simulink model "CranePID1"  (Simulink 5.0)
settings: Solver=ode5  SolverMode=SingleTasking  StartTime=0.0  StopTime=50.0  FixedStep=0.001  RelTol=1e-3
libraries: pci1711 x3
settings Model: LastModifiedBy=cedrics  ExtModeMexFile=rtwinext  ExtModeTrigMode=oneshot  ExtModeTrigDuration=100000  ExtModeLogAll=off  SimulationMode=external  LimitDataPoints=off  BlockReductionOpt=off  BooleanDataType=off  RTWSystemTargetFile=rtwinfbk.tlc  RTWTemplateMakefile=winfbktmf  RTWOptions="-aCCOptimize=1 -aEnforceIntegerDowncast=1 -aExtMode=1 -aFoldNonRolledExpr=1 -aForceParamTrailComments=0 -aGenerateComments=1 -aGenerateReport=0 -aIncDataTypeInIds=0 -aIncHierarchyInIds=0 -aInlineInvariantSignals=0 -aInlineParameters=0 -aInlinedPrmAccess=\"Literals\" -aLocalBlockOutputs=1 -aMaxRTWIdLen=31 -aPrefixModelToSubsysFcnNames=1 -aRTWVerbose=1 -aRebuildAll=0 -aRollThreshold=5 -aShowEliminatedStatements=1"

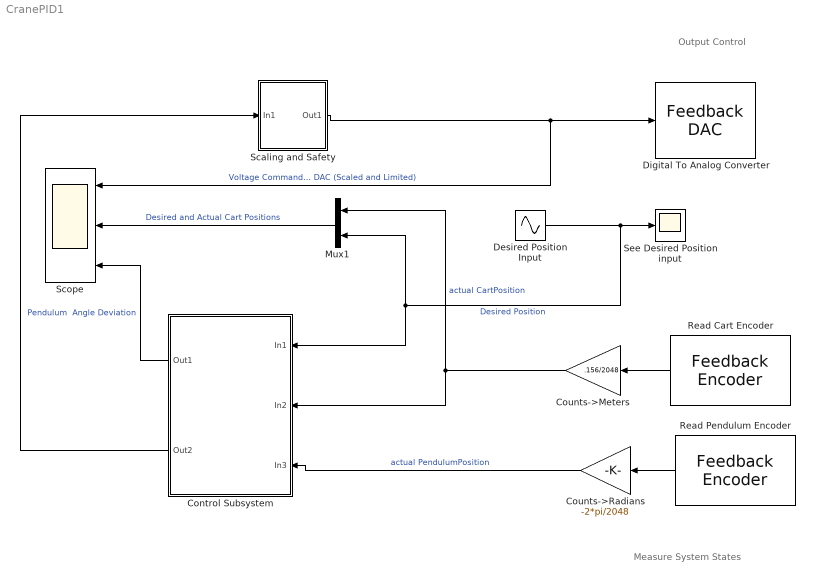
== system CranePID1 ==
  note: Measure System States
  note: Output Control
  Control Subsystem : Subsystem  Orientation=left
  Counts->Meters : Gain  Orientation=left  Gain=.156/2048  SaturateOnIntegerOverflow=on
  Counts->Radians : Gain  Orientation=left  Gain=-2*pi/2048  SaturateOnIntegerOverflow=on
  Desired Position Input : Sin  Amplitude=0.2  SampleTime=0
  "Digital To Analog Converter " : pci1711/Advantech  PCI1711 I//O Board Lib/Feedback DAC  channel=0  range=0  tsamp=0.001  hwAccess=on
  Mux1 : Mux  Orientation=left  Inputs=2
  Read Cart Encoder : pci1711/Advantech  PCI1711 I//O Board Lib/Feedback Encoder   Orientation=left  channel=0  offset=0  tsamp=0.001  hwAccess=on
  Read Pendulum Encoder : pci1711/Advantech  PCI1711 I//O Board Lib/Feedback Encoder   Orientation=left  channel=1  offset=-1024  tsamp=0.001  hwAccess=on
  Scaling and Safety : Subsystem
  Scope : Scope  NumInputPorts=3
      settings: TickLabels=on  TimeRange=50  YMin=-2.5~-0.3~-3.5  YMax=2.5~0.3~3.5  Decimation=10  SampleInput=on  SampleTime=0.01
  See Desired Position input : Scope
      settings: YMin=-0.75  YMax=1.5  SampleInput=on  SampleTime=0.1
  wires:
  Read Cart Encoder/1 -> Counts->Meters/1
  Counts->Meters/1 -> Mux1/1, Control Subsystem/2(In2)  "actual CartPosition"
  Counts->Radians/1 -> Control Subsystem/3(In3)  "actual PendulumPosition"
  Control Subsystem/2(Out2) -> Scaling and Safety/1(In1)
  Mux1/1 -> Scope/2  "Desired and Actual Cart Positions"
  Control Subsystem/1(Out1) -> Scope/3  "Pendulum  Angle Deviation"
  Read Pendulum Encoder/1 -> Counts->Radians/1
  Scaling and Safety/1(Out1) -> Scope/1, "Digital To Analog Converter "/1  "Voltage Command to DAC (Scaled and Limited)"
  Desired Position Input/1 -> Mux1/2, Control Subsystem/1(In1), See Desired Position input/1  "Desired Position"

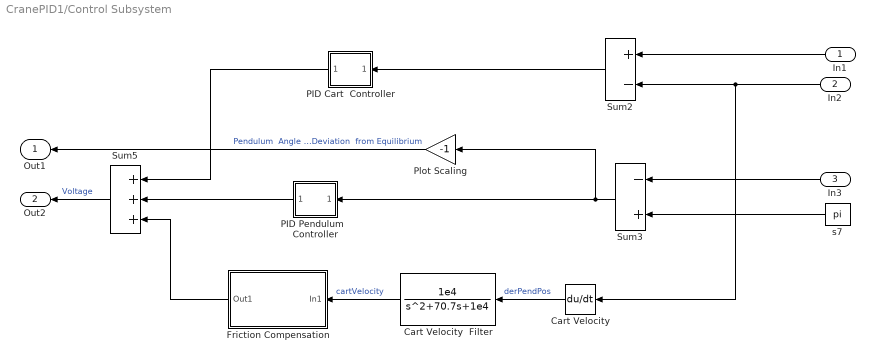
== system CranePID1/Control Subsystem ==
  In1 : Inport  Orientation=left
  In2 : Inport  Orientation=left  Port=2
  In3 : Inport  Orientation=left  Port=3
  Cart Velocity : Derivative  Orientation=left
  Cart Velocity  Filter : TransferFcn  Orientation=left  Numerator=[1e4]  Denominator=[1 70.7 1e4]
  Friction Compensation : Subsystem  Orientation=left  mask(linear){frictionCompNeg=.1, frictionCompPos=.1}
      mask prompts: frictionCompNeg "Friction Compensation Magnitude in Negative Direction"; frictionCompPos "Friction Compensation Magnitude in Positive Direction"
      mask Display: plot(0,0,100,100,[40,30,20],[87,85,80],[46,54,54,46,46],[90,90,80,80,90],[46,45,45,46,54,55,55,54,46],[78,80,90,91,91,90,80,78,78],[51,51,49,49],[78,10,10,78],[90,80,70,60],[70,80,85,88],[20,10],[80,70],[20,20,15],[73,80,80],[85,80,80],[80,80,74])
  PID Cart  Controller : Subsystem  Orientation=left  mask(PID Controller){@1=10, @2=1, @3=2}
      mask prompts: @1 "Proportional:"; @2 "Integral"; @3 "Derivative:"
      mask help:
      | Enter expressions for proportional, integral, and derivative terms.
      | P+I/s+Ds
      mask init:
      | P=@1; I=@2; D=@3;
      mask Help: This block implements a PID controller where parameters are entered for the Proportional, Integral and Derivative terms. Unmask this block to see how it works. The derivative term is implemented using a true derivative block.
      mask Display: disp('PID')
  PID Pendulum   Controller : Subsystem  Orientation=left  mask(PID Controller){@1=-5, @2=0, @3=0}
      mask prompts: @1 "Proportional:"; @2 "Integral"; @3 "Derivative:"
      mask help:
      | Enter expressions for proportional, integral, and derivative terms.
      | P+I/s+Ds
      mask init:
      | P=@1; I=@2; D=@3;
      mask Help: This block implements a PID controller where parameters are entered for the Proportional, Integral and Derivative terms. Unmask this block to see how it works. The derivative term is implemented using a true derivative block.
      mask Display: disp('PID')
  Plot Scaling : Gain  Orientation=left  Gain=-1  SaturateOnIntegerOverflow=on
  Sum2 : Sum  Orientation=left  Inputs=+-  SaturateOnIntegerOverflow=on  InputSameDT=on
  Sum3 : Sum  Orientation=left  Inputs=-+  SaturateOnIntegerOverflow=on  InputSameDT=on
  Sum5 : Sum  Orientation=left  Inputs=+++  SaturateOnIntegerOverflow=on  InputSameDT=on
  s7 : Constant  Orientation=left  Value=pi
  Out1 : Outport  Orientation=left
  Out2 : Outport  Orientation=left  Port=2
  wires:
  s7/1 -> Sum3/2
  Sum2/1 -> PID Cart  Controller/1(In_1)
  Cart Velocity  Filter/1 -> Friction Compensation/1(In1)  "cartVelocity"
  Cart Velocity/1 -> Cart Velocity  Filter/1  "derPendPos"
  PID Pendulum   Controller/1(Out_1) -> Sum5/2
  Friction Compensation/1(Out1) -> Sum5/3
  PID Cart  Controller/1(Out_1) -> Sum5/1
  Sum3/1 -> PID Pendulum   Controller/1(In_1), Plot Scaling/1
  In1/1 -> Sum2/1
  In2/1 -> Sum2/2, Cart Velocity/1
  Plot Scaling/1 -> Out1/1  "Pendulum  Angle Deviation  from Equilibrium"
  In3/1 -> Sum3/1
  Sum5/1 -> Out2/1  "Voltage"

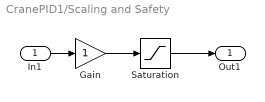
== system CranePID1/Scaling and Safety ==
  In1 : Inport
  Gain : Gain  SaturateOnIntegerOverflow=on
  Saturation : Saturate  UpperLimit=2.5  LowerLimit=-2.5
  Out1 : Outport
  wires:
  Saturation/1 -> Out1/1
  In1/1 -> Gain/1
  Gain/1 -> Saturation/1

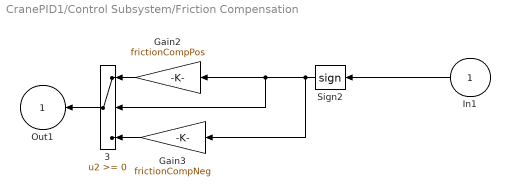
== system CranePID1/Control Subsystem/Friction Compensation ==
  In1 : Inport  Orientation=left
  3 : Switch  Orientation=left  SaturateOnIntegerOverflow=on  InputSameDT=on
  Gain2 : Gain  Orientation=left  Gain=frictionCompPos  SaturateOnIntegerOverflow=on
  Gain3 : Gain  Orientation=left  Gain=frictionCompNeg  SaturateOnIntegerOverflow=on
  Sign2 : Signum  Tag=T  Orientation=left
  Out1 : Outport  Orientation=left  InitialOutput=0
  wires:
  3/1 -> Out1/1
  Sign2/1 -> 3/2, Gain2/1, Gain3/1
  Gain3/1 -> 3/3
  Gain2/1 -> 3/1
  In1/1 -> Sign2/1

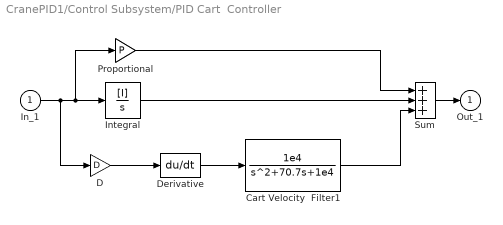
== system CranePID1/Control Subsystem/PID Cart  Controller ==
  In_1 : Inport
  Cart Velocity  Filter1 : TransferFcn  Numerator=[1e4]  Denominator=[1 70.7 1e4]
  D : Gain  Gain=D  SaturateOnIntegerOverflow=on
  Derivative : Derivative
  Integral : TransferFcn  Numerator=[I]  Denominator=[1 0]
  Proportional : Gain  Gain=P  SaturateOnIntegerOverflow=on
  Sum : Sum  Inputs=+++  SaturateOnIntegerOverflow=on  InputSameDT=on
  Out_1 : Outport  InitialOutput=0
  wires:
  In_1/1 -> Integral/1, Proportional/1, D/1
  Proportional/1 -> Sum/1
  Integral/1 -> Sum/2
  Sum/1 -> Out_1/1
  D/1 -> Derivative/1
  Derivative/1 -> Cart Velocity  Filter1/1
  Cart Velocity  Filter1/1 -> Sum/3

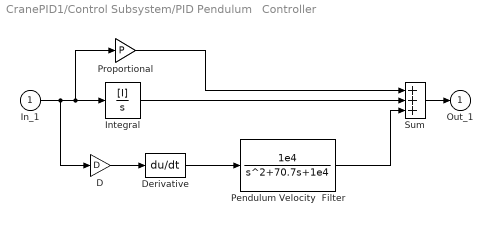
== system CranePID1/Control Subsystem/PID Pendulum   Controller ==
  In_1 : Inport
  D : Gain  Gain=D  SaturateOnIntegerOverflow=on
  Derivative : Derivative
  Integral : TransferFcn  Numerator=[I]  Denominator=[1 0]
  Pendulum Velocity  Filter : TransferFcn  Numerator=[1e4]  Denominator=[1 70.7 1e4]
  Proportional : Gain  Gain=P  SaturateOnIntegerOverflow=on
  Sum : Sum  Inputs=+++  SaturateOnIntegerOverflow=on  InputSameDT=on
  Out_1 : Outport  InitialOutput=0
  wires:
  D/1 -> Derivative/1
  In_1/1 -> D/1, Integral/1, Proportional/1
  Integral/1 -> Sum/2
  Proportional/1 -> Sum/1
  Sum/1 -> Out_1/1
  Derivative/1 -> Pendulum Velocity  Filter/1
  Pendulum Velocity  Filter/1 -> Sum/3
